simulink library "meaworklibrary"  (Simulink 6.5)
libraries: meaworklibrary x6, simulink x1
settings Model: Creator=Marom  LastModifiedBy=Marom

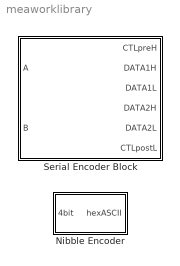
== system meaworklibrary ==
  Nibble Encoder : Subsystem
      mask Description: encodes 4-element binary (uint8) vector (most significant first) to hexASCII representation (unit8)
  Serial Encoder Block : Subsystem
      mask Description: encodes two 8 element vector A and B boolean signals (unit8) for MEA Serial Port

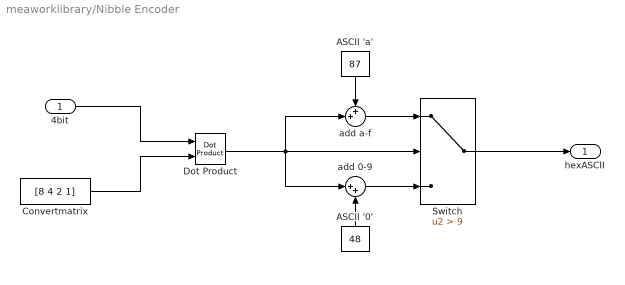
== system meaworklibrary/Nibble Encoder ==
  4bit : Inport  PortDimensions=4  DataType=uint8
  ASCII '0' : Constant  Orientation=up  Value=48  OutDataTypeMode=uint8  OutDataType=sfix(16)  ConRadixGroup=Use specified scaling  OutScaling=2^0  SampleTime=inf  FramePeriod=inf
  ASCII 'a' : Constant  Orientation=down  Value=87  OutDataTypeMode=uint8  OutDataType=sfix(16)  ConRadixGroup=Use specified scaling  OutScaling=2^0  SampleTime=inf  FramePeriod=inf
  Convertmatrix : Constant  Value=[8 4 2 1]  OutDataTypeMode=uint8  OutDataType=sfix(16)  ConRadixGroup=Use specified scaling  OutScaling=2^0  SampleTime=inf  FramePeriod=inf
  Dot Product : simulink/Math Operations/Dot Product  InputSameDT=on  OutDataType=sfix(16)  OutScaling=2^-10  DoSatur=off
  Switch : Switch  Criteria=u2 > Threshold  Threshold=9
  add 0-9 : Sum  Inputs=|++  OutDataTypeMode=uint8  OutScaling=2^-10
  add a-f : Sum  Inputs=++|  OutDataTypeMode=uint8  OutScaling=2^-10
  hexASCII : Outport  DataType=uint8
  wires:
  Switch/1 -> hexASCII/1
  add 0-9/1 -> Switch/3
  ASCII '0'/1 -> add 0-9/2
  ASCII 'a'/1 -> add a-f/1
  add a-f/1 -> Switch/1
  Dot Product/1 -> Switch/2, add 0-9/1, add a-f/2
  Convertmatrix/1 -> Dot Product/2
  4bit/1 -> Dot Product/1

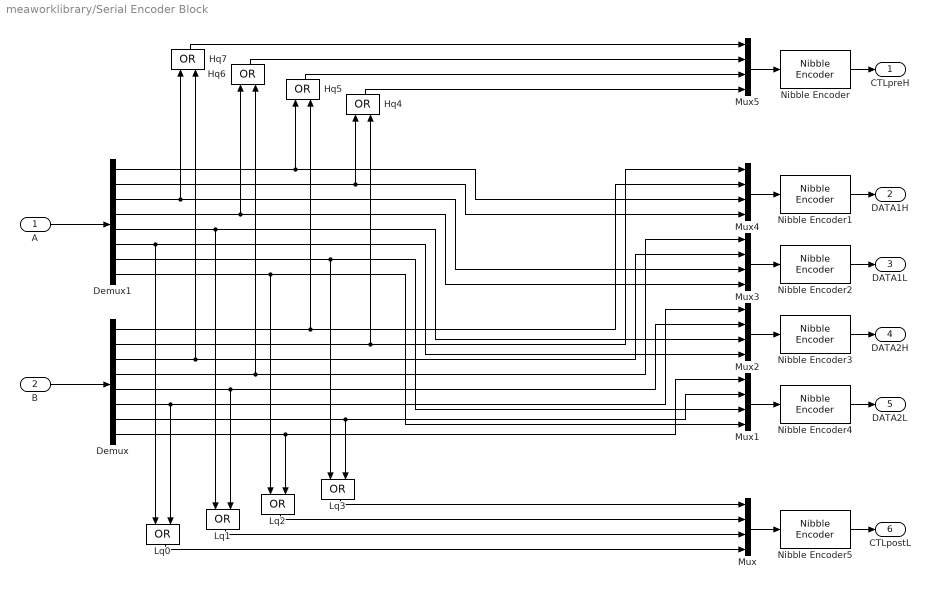
== system meaworklibrary/Serial Encoder Block ==
  A : Inport  PortDimensions=8
  B : Inport  Port=2  PortDimensions=8
  Demux : Demux  Outputs=8
  Demux1 : Demux  Outputs=8
  Hq{4..7} (4 alike) : Logic  Orientation=up  Operator=OR  AllPortsSameDT=off  OutDataTypeMode=Specify via dialog
  Lq{0..3} (4 alike) : Logic  Orientation=down  Operator=OR  AllPortsSameDT=off  OutDataTypeMode=Specify via dialog
  Mux{,1..5} (6 alike) : Mux
  Nibble Encoder{,1..5} (6 alike) : meaworklibrary/Nibble Encoder  SystemSampleTime=-1
  CTLpreH : Outport  DataType=uint8
  DATA1H : Outport  Port=2  DataType=uint8
  DATA1L : Outport  Port=3  DataType=uint8
  DATA2H : Outport  Port=4  DataType=uint8
  DATA2L : Outport  Port=5  DataType=uint8
  CTLpostL : Outport  Port=6  DataType=uint8
  wires:
  Nibble Encoder3/1 -> DATA2H/1
  Mux2/1 -> Nibble Encoder3/1
  Mux3/1 -> Nibble Encoder2/1
  Nibble Encoder2/1 -> DATA1L/1
  Lq0/1 -> Mux/4
  Lq1/1 -> Mux/3
  Lq2/1 -> Mux/2
  Lq3/1 -> Mux/1
  Hq7/1 -> Mux5/1
  Hq6/1 -> Mux5/2
  Hq4/1 -> Mux5/4
  Hq5/1 -> Mux5/3
  Nibble Encoder/1 -> CTLpreH/1
  Nibble Encoder5/1 -> CTLpostL/1
  Nibble Encoder4/1 -> DATA2L/1
  Mux5/1 -> Nibble Encoder/1
  Mux/1 -> Nibble Encoder5/1
  Mux1/1 -> Nibble Encoder4/1
  Nibble Encoder1/1 -> DATA1H/1
  Mux4/1 -> Nibble Encoder1/1
  Demux/8 -> Lq2/2, Mux1/1
  Demux/7 -> Lq3/2, Mux1/2
  Demux/6 -> Lq0/2, Mux2/1
  Demux/5 -> Lq1/2, Mux2/2
  Demux/4 -> Hq6/2, Mux3/1
  Demux/3 -> Hq7/2, Mux3/2
  Demux/2 -> Hq4/2, Mux4/1
  Demux/1 -> Hq5/2, Mux4/2
  Demux1/8 -> Lq2/1, Mux1/4
  Demux1/7 -> Lq3/1, Mux1/3
  Demux1/6 -> Lq0/1, Mux2/4
  Demux1/5 -> Lq1/1, Mux2/3
  Demux1/4 -> Hq6/1, Mux3/4
  Demux1/3 -> Hq7/1, Mux3/3
  Demux1/2 -> Hq4/1, Mux4/4
  Demux1/1 -> Hq5/1, Mux4/3
  A/1 -> Demux1/1
  B/1 -> Demux/1
